simulink model "FuzzyPersonalizableDMA"  (R2024b)
settings: Solver=ode45  StartTime=0.0  StopTime=3  FixedStep=.1  RelTol=1e-3
libraries: fuzblock x1
settings Model: Creator=aceve  LastModifiedBy=david

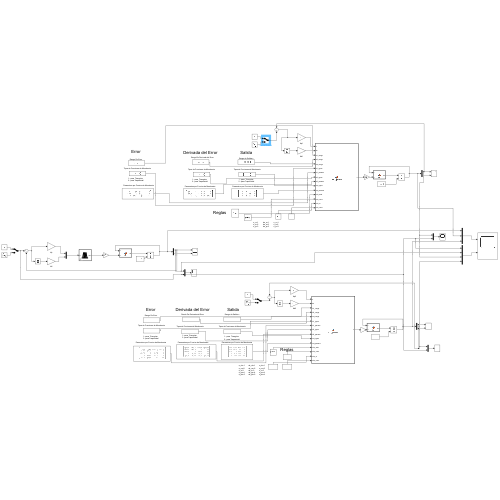
[thumbnail: Simulink's stored preview of the top-level diagram]
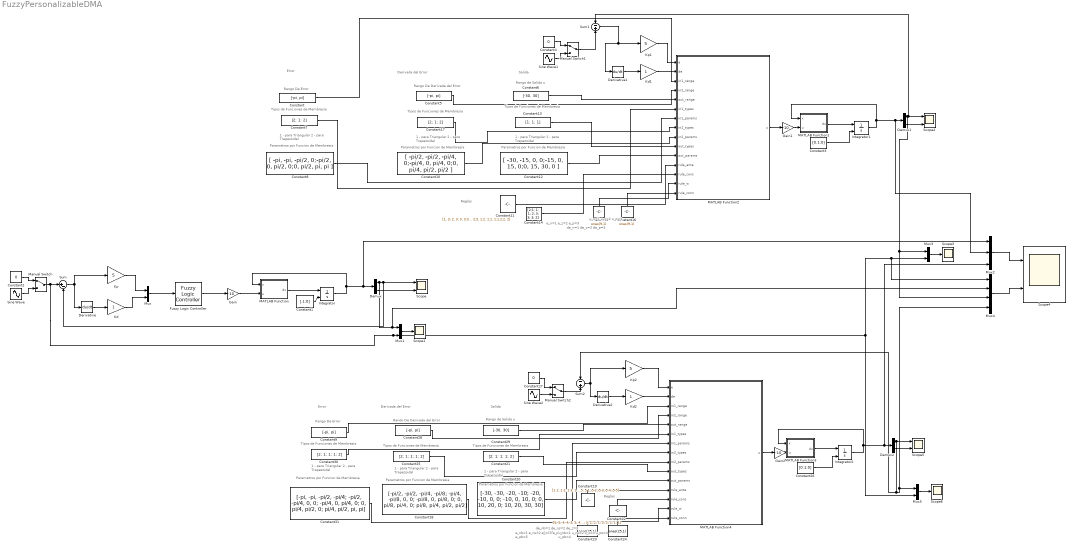
== system FuzzyPersonalizableDMA ==
  note: e_n=1
      | e_z=2
      | e_p=3
  note: Error
  note: 1 - para  Triangular
      | 2 - para Trapezoidal
  note: Parametros por Funcion de Membresia
  note: Tipos de Funciones de Membresia
  note: Rango de Salida u
  note: Rango De Derivada del Error
  note: Rango De Error
  note: 1 - para  Triangular
      | 2 - para Trapezoidal
  note: Derivada del Error
  note: Tipos de Funciones de Membresia
  note: Parametros por Funcion de Membresia
  note: 1 - para  Triangular
      | 2 - para Trapezoidal
  note: Salida
  note: Tipos de Funciones de Membresia
  note: Parametros por Funcion de Membresia
  note: Reglas
  note: de_n=1
      | de_z=2
      | de_p=3
  note: u_n=1
      | u_z=2
      | u_p=3
  note: 1 - para  Triangular
      | 2 - para Trapezoidal
  note: Tipos de Funciones de Membresia
  note: Salida
  note: de_nb=1
      | de_ns=2
      | de_z=3
      | de_ps=4
      | de_pb=5
  note: Reglas
  note: Parametros por Funcion de Membresia
  note: e_nb=1
      | e_ns=2
      | e_z=3
      | e_ps=4
      | e_pb=5
  note: Rando De Derivada del Error
  note: Error
  note: 1 - para  Triangular
      | 2 - para Trapezoidal
  note: Tipos de Funciones de Membresia
  note: Rango De Error
  note: Parametros por Funcion de Membresia
  note: Parametros por Funcion de Membresia
  note: u_nb=1
      | u_ns=2
      | u_z=3
      | u_ps=4
      | u_pb=4
  note: Tipos de Funciones de Membresia
  note: 1 - para  Triangular
      | 2 - para Trapezoidal
  note: Rango de Salida u
  note: Derivada del Error
  Constant{,5,9,28} (4 alike) : Constant  Value=[-pi, pi]
  Constant1 : Constant  Value=[.1;0]
  Constant10 : Constant  Value=[ -pi/2, -pi/2, -pi/4, 0;-pi/4, 0, pi/4, 0;0, pi/4, pi/2, pi/2 ]
  Constant11 : Constant  Value=[1, 3; 2, 3; 3, 3;3, 2;3, 1;2, 1;1, 1;1,2;2, 2]
  Constant12 : Constant  Value="[ -30, -15, 0, 0;-15,   0, 15, 0;0,  15, 30, 0 ]"
  Constant13 : Constant  Value=[1; 1; 1]
  Constant14 : Constant  Value=[2;1; 1; 1; 2; 3; 3; 3; 2]
  Constant15 : Constant  Value=ones(9,1)
  Constant16 : Constant  Value=ones(9,1)
  Constant17 : Constant  Value=[2; 1; 2]
  Constant18 : Constant  Value=[-pi/2, -pi/2, -pi/4, -pi/8; -pi/4, -pi/8, 0, 0; -pi/8, 0, pi/8, 0; 0, pi/8, pi/4, 0; pi/8, pi/4, pi/2, pi/2]
  Constant19 : Constant  Value=[1 1; 1 2; 1 3; 1 4; 1 5; 2 1; 2 2; 2 3; 2 4; 2 5; 3 1; 3 2; 3 3; 3 4; 3 5; 4 1; 4 2; 4 3; 4 4; 4 5; 5 1; 5 2; 5 3; 5 4; 5 5]
  Constant2 : Constant  Value=0
  Constant20 : Constant  Value=[-30, -30, -20, -10; -20, -10, 0, 0; -10, 0, 10, 0; 0, 10, 20, 0; 10, 20, 30, 30]
  Constant21 : Constant  Value=[2; 1; 1; 1; 2]
  Constant22 : Constant  Value=[5; 5; 4; 4; 3; 5; 4; 4; 3; 2; 4; 4; 3; 2; 2; 4; 3; 2; 2; 1; 3; 2; 2; 1; 1]
  Constant23 : Constant  Value=ones(25,1)
  Constant24 : Constant  Value=ones(25,1)
  Constant25 : Constant  Value=[2; 1; 1; 1; 2]
  Constant26 : Constant  Value=[0.1;0]
  Constant27 : Constant  Value=0
  Constant29 : Constant  Value=[-30, 30]
  Constant3 : Constant  Value=[0.1;0]
  Constant30 : Constant  Value=[2; 1; 1; 1; 2]
  Constant31 : Constant  Value=[-pi, -pi, -pi/2, -pi/4; -pi/2, -pi/4, 0, 0; -pi/4, 0, pi/4, 0; 0, pi/4, pi/2, 0; pi/4, pi/2, pi, pi]
  Constant4 : Constant  Value=0
  Constant6 : Constant  Value=[-30, 30]
  Constant7 : Constant  Value=[2; 1; 2]
  Constant8 : Constant  Value=[ -pi, -pi, -pi/2, 0;-pi/2, 0, pi/2, 0;0, pi/2, pi, pi ]
  Demux : Demux  Outputs=2
  Demux1 : Demux  Outputs=2
  Demux2 : Demux  Outputs=2
  Derivative : Derivative
  Derivative1 : Derivative
  Derivative2 : Derivative
  Fuzzy Logic Controller : fuzblock/Fuzzy Logic  Controller  FIS='3x3man.fis'  OutputSampleNumber=101  DataType=double  FuzzifiedInputs=off  RuleFiringStrengths=off  RuleOutputs=off  AggregatedOutputs=off  SimulateUsing=Interpreted execution  OutOfRangeInputValueMessage=warning  NoRuleFiredMessage=warning  EmptyOutputFuzzySetMessage=warning
  Gain : Gain  Gain=-10
  Gain1 : Gain  Gain=-10
  Gain2 : Gain  Gain=-10
  Integrator : Integrator  InitialConditionSource=external
  Integrator1 : Integrator  InitialConditionSource=external
  Integrator2 : Integrator  InitialConditionSource=external
  Kd : Gain
  Kd1 : Gain
  Kd2 : Gain
  Kp : Gain  Gain=5
  Kp1 : Gain  Gain=5
  Kp2 : Gain  Gain=5
  MATLAB Function : MATLAB Function  TreatAsAtomicUnit=on
  MATLAB Function1 : MATLAB Function  TreatAsAtomicUnit=on
  MATLAB Function2 : MATLAB Function  TreatAsAtomicUnit=on
  MATLAB Function3 : MATLAB Function  TreatAsAtomicUnit=on
  MATLAB Function4 : MATLAB Function  TreatAsAtomicUnit=on
  Manual Switch : ManualSwitch
  Manual Switch1 : ManualSwitch
  Manual Switch2 : ManualSwitch
  Mux{,1,3,5} (4 alike) : Mux  Inputs=2
  Mux2 : Mux  Inputs=3
  Mux4 : Mux
  Scope{,2,4..5} (4 alike) : Scope  NumInputPorts=2
  Scope1 : Scope
  Scope3 : Scope
  Scope6 : Scope
  Sine Wave : Sin  Amplitude=.25  Frequency=4  SampleTime=0
  Sine Wave1 : Sin  Amplitude=.25  Frequency=4  SampleTime=0
  Sine Wave2 : Sin  Amplitude=.25  Frequency=4  SampleTime=0
  Sum : Sum  Inputs=|+-
  Sum1 : Sum  Inputs=-|+
  Sum2 : Sum  Inputs=-|+
  wires:
  Integrator/1 -> MATLAB Function/1(x), Mux2/1, Demux/1
  Demux/1 -> Scope/1, Sum/2, Mux4/2, Mux1/1
  Demux/2 -> Scope/2
  Constant1/1 -> Integrator/2
  Fuzzy Logic Controller/1 -> Gain/1
  Gain/1 -> MATLAB Function/2(u)
  Mux/1 -> Fuzzy Logic Controller/1
  Kp/1 -> Mux/1
  Constant2/1 -> Manual Switch/1
  Sine Wave/1 -> Manual Switch/2
  Sum/1 -> Derivative/1, Kp/1
  Kd/1 -> Mux/2
  Derivative/1 -> Kd/1
  Mux1/1 -> Scope1/1
  MATLAB Function/1(dx) -> Integrator/1
  Sine Wave1/1 -> Manual Switch1/2
  Constant4/1 -> Manual Switch1/1
  Demux1/2 -> Scope2/2
  Demux1/1 -> Scope2/1, Sum1/1, Mux4/3, Mux3/1
  MATLAB Function1/1(dx) -> Integrator1/1
  Integrator1/1 -> MATLAB Function1/1(x), Mux2/2, Demux1/1
  Gain1/1 -> MATLAB Function1/2(u)
  Constant3/1 -> Integrator1/2
  Mux3/1 -> Scope3/1
  Derivative1/1 -> Kd1/1
  Mux2/1 -> Scope4/1
  Mux4/1 -> Scope4/2
  MATLAB Function2/1(u) -> Gain1/1
  Manual Switch1/1 -> Sum1/2
  Sum1/1 -> Derivative1/1, Kp1/1
  Constant/1 -> MATLAB Function2/3(in1_range)
  Constant5/1 -> MATLAB Function2/4(in2_range)
  Constant6/1 -> MATLAB Function2/5(out_range)
  Constant7/1 -> MATLAB Function2/6(in1_types)
  Constant8/1 -> MATLAB Function2/7(in1_params)
  Constant17/1 -> MATLAB Function2/8(in2_types)
  Constant13/1 -> MATLAB Function2/10(out_types)
  Constant12/1 -> MATLAB Function2/11(out_params)
  Manual Switch/1 -> Mux1/2, Mux5/2, Mux4/1, Mux3/2, Sum/1
  Constant16/1 -> MATLAB Function2/15(rule_conn)
  Constant15/1 -> MATLAB Function2/14(rule_w)
  Constant14/1 -> MATLAB Function2/13(rule_cons)
  Constant11/1 -> MATLAB Function2/12(rule_ante)
  Constant21/1 -> MATLAB Function4/10(out_types)
  Constant23/1 -> MATLAB Function4/14(rule_w)
  Derivative2/1 -> Kd2/1
  Constant26/1 -> Integrator2/2
  Mux5/1 -> Scope6/1
  Constant25/1 -> MATLAB Function4/8(in2_types)
  Sum2/1 -> Derivative2/1, Kp2/1
  MATLAB Function4/1(u) -> Gain2/1
  Constant9/1 -> MATLAB Function4/3(in1_range)
  Constant30/1 -> MATLAB Function4/6(in1_types)
  Manual Switch2/1 -> Sum2/2
  Gain2/1 -> MATLAB Function3/2(u)
  MATLAB Function3/1(dx) -> Integrator2/1
  Constant29/1 -> MATLAB Function4/5(out_range)
  Sine Wave2/1 -> Manual Switch2/2
  Constant22/1 -> MATLAB Function4/13(rule_cons)
  Constant18/1 -> MATLAB Function4/9(in2_params)
  Constant31/1 -> MATLAB Function4/7(in1_params)
  Integrator2/1 -> MATLAB Function3/1(x), Mux2/3, Demux2/1
  Constant24/1 -> MATLAB Function4/15(rule_conn)
  Constant19/1 -> MATLAB Function4/12(rule_ante)
  Constant20/1 -> MATLAB Function4/11(out_params)
  Demux2/1 -> Mux5/1, Mux4/4, Sum2/1, Scope5/1
  Demux2/2 -> Scope5/2
  Constant27/1 -> Manual Switch2/1
  Constant28/1 -> MATLAB Function4/4(in2_range)
  Kd2/1 -> MATLAB Function4/2(de)
  Kp2/1 -> MATLAB Function4/1(e)
  Kd1/1 -> MATLAB Function2/2(de)
  Kp1/1 -> MATLAB Function2/1(e)
  Constant10/1 -> MATLAB Function2/9(in2_params)

== matlab function FuzzyPersonalizableDMA/MATLAB Function1 ==
  data: x input; dx output; u input
function dx  = fcn(x,u)

l = 1;
m = 1;
g = 9.81;
b = 0.5;
I = m*l^2

x1 = x(1);
x2 = x(2);
dx1 = x2;
dx2 = g/l * sin(x1) - b*l/I * x2 + u/I;
dx = [dx1;dx2];

y = u;

== matlab function FuzzyPersonalizableDMA/MATLAB Function ==
  data: x input; dx output; u input
function dx  = fcn(x,u)

l = 1;
m = 1;
g = 9.81;
b = 0.5;
I = m*l^2

x1 = x(1);
x2 = x(2);
dx1 = x2;
dx2 = g/l * sin(x1) - b*l/I * x2 + u/I;
dx = [dx1;dx2];

y = u;

== matlab function FuzzyPersonalizableDMA/MATLAB Function2 ==
  data: e input; u output; de input; in1_range input; in2_range input; out_range input; in1_types input; in1_params input; in2_types input; in2_params input; out_types input; out_params input; rule_ante input; rule_cons input; rule_w input; rule_conn input
function u = FLC_generic(e, de, ...
    in1_range, in2_range, out_range, ...
    in1_types, in1_params, ...   % [N1x1], [N1x4]
    in2_types, in2_params, ...   % [N2x1], [N2x4]
    out_types, out_params, ...   % [N3x1], [N3x4]
    rule_ante, rule_cons, rule_w, rule_conn)
%#codegen
% Mamdani: AND=min, OR=max, Imp=min, Agg=max, Defuzz=centroid
% Tipos: 1=trimf (usa a,b,c en cols 1..3), 2=trapmf (usa a,b,c,d en 1..4)
% rule_ante: [R x 2] índices de MF para [e, de] (0 = "no importa")
% rule_cons: [R x 1] índice de MF de salida
% rule_w:    [R x 1] peso en [0,1]
% rule_conn: [R x 1] 1=AND(min) 2=OR(max)  (aquí solo 1 o 2)

% ---- fuzzificación entradas ----
N1 = numel(in1_types);
N2 = numel(in2_types);
muE  = zeros(1,N1);
muDE = zeros(1,N2);
for i=1:N1
    muE(i) = mf_eval(e, in1_types(i), in1_params(i,:));
end
for j=1:N2
    muDE(j) = mf_eval(de, in2_types(j), in2_params(j,:));
end

% ---- inferencia (implicación min) y agregación (max) ----
Nout = numel(out_types);
% Universo de discurso de salida
Nu = 301;
ug = linspace(out_range(1), out_range(2), Nu);
muAgg = zeros(1,Nu);

R = size(rule_ante,1);
for r = 1:R
    i = rule_ante(r,1);  % MF index para e  (0=DC)
    j = rule_ante(r,2);  % MF index para de (0=DC)
    k = rule_cons(r);    % MF index salida
    w = rule_w(r);       % peso
    conn = rule_conn(r); % 1=min, 2=max

    % firing strength del antecedente
    a1 = 1.0; if i>0, a1 = muE(i);  end
    a2 = 1.0; if j>0, a2 = muDE(j); end
    if conn==1       % AND=min
        alpha = min(a1,a2);
    else             % OR=max
        alpha = max(a1,a2);
    end
    alpha = max(0,min(1, alpha*w));

    if alpha<=0 || k<1 || k>Nout
        continue
    end

    % MF de salida recortada por alpha: mu_k_out = min(alpha, mf_out)
    mu_k = zeros(1,Nu);
    for t=1:Nu
        mu_k(t) = mf_eval(ug(t), out_types(k), out_params(k,:));
    end
    muAgg = max(muAgg, min(alpha, mu_k));
end

% ---- desdifusificación (centroide) ----
num = sum(ug .* muAgg);
den = sum(muAgg);
if den<=eps
    % sin activación: salida neutra dentro de rango
    u = 0.5*(out_range(1)+out_range(2));
else
    u = num/den;
end
end

% ================= helpers =================
function mu = mf_eval(x, type_id, p)
% p es 1x4, usa solo los necesarios
if type_id==1 % trimf [a b c]
    a=p(1); b=p(2); c=p(3);
    if x<=a || x>=c, mu=0;
    elseif x==b, mu=1;
    elseif x>a && x<b, mu=(x-a)/max(b-a,eps);
    else, mu=(c-x)/max(c-b,eps);
    end
elseif type_id==2 % trapmf [a b c d]
    a=p(1); b=p(2); c=p(3); d=p(4);
    if x<=a || x>=d, mu=0;
    elseif x>=b && x<=c, mu=1;
    elseif x>a && x<b,  mu=(x-a)/max(b-a,eps);
    else                mu=(d-x)/max(d-c,eps);
    end
else
    mu = 0; % tipo desconocido
end
end

== matlab function FuzzyPersonalizableDMA/MATLAB Function3 ==
  data: x input; dx output; u input
function dx  = fcn(x,u)

l = 1;
m = 1;
g = 9.81;
b = 0.5;
I = m*l^2

x1 = x(1);
x2 = x(2);
dx1 = x2;
dx2 = g/l * sin(x1) - b*l/I * x2 + u/I;
dx = [dx1;dx2];

y = u;

== matlab function FuzzyPersonalizableDMA/MATLAB Function4 ==
  data: e input; u output; de input; in1_range input; in2_range input; out_range input; in1_types input; in1_params input; in2_types input; in2_params input; out_types input; out_params input; rule_ante input; rule_cons input; rule_w input; rule_conn input
function u = FLC_generic(e, de, ...
    in1_range, in2_range, out_range, ...
    in1_types, in1_params, ...   % [N1x1], [N1x4]
    in2_types, in2_params, ...   % [N2x1], [N2x4]
    out_types, out_params, ...   % [N3x1], [N3x4]
    rule_ante, rule_cons, rule_w, rule_conn)
%#codegen
% Mamdani: AND=min, OR=max, Imp=min, Agg=max, Defuzz=centroid
% Tipos: 1=trimf (usa a,b,c en cols 1..3), 2=trapmf (usa a,b,c,d en 1..4)
% rule_ante: [R x 2] índices de MF para [e, de] (0 = "no importa")
% rule_cons: [R x 1] índice de MF de salida
% rule_w:    [R x 1] peso en [0,1]
% rule_conn: [R x 1] 1=AND(min) 2=OR(max)  (aquí solo 1 o 2)

% ---- fuzzificación entradas ----
N1 = numel(in1_types);
N2 = numel(in2_types);
muE  = zeros(1,N1);
muDE = zeros(1,N2);
for i=1:N1
    muE(i) = mf_eval(e, in1_types(i), in1_params(i,:));
end
for j=1:N2
    muDE(j) = mf_eval(de, in2_types(j), in2_params(j,:));
end

% ---- inferencia (implicación min) y agregación (max) ----
Nout = numel(out_types);
% Universo de discurso de salida
Nu = 301;
ug = linspace(out_range(1), out_range(2), Nu);
muAgg = zeros(1,Nu);

R = size(rule_ante,1);
for r = 1:R
    i = rule_ante(r,1);  % MF index para e  (0=DC)
    j = rule_ante(r,2);  % MF index para de (0=DC)
    k = rule_cons(r);    % MF index salida
    w = rule_w(r);       % peso
    conn = rule_conn(r); % 1=min, 2=max

    % firing strength del antecedente
    a1 = 1.0; if i>0, a1 = muE(i);  end
    a2 = 1.0; if j>0, a2 = muDE(j); end
    if conn==1       % AND=min
        alpha = min(a1,a2);
    else             % OR=max
        alpha = max(a1,a2);
    end
    alpha = max(0,min(1, alpha*w));

    if alpha<=0 || k<1 || k>Nout
        continue
    end

    % MF de salida recortada por alpha: mu_k_out = min(alpha, mf_out)
    mu_k = zeros(1,Nu);
    for t=1:Nu
        mu_k(t) = mf_eval(ug(t), out_types(k), out_params(k,:));
    end
    muAgg = max(muAgg, min(alpha, mu_k));
end

% ---- desdifusificación (centroide) ----
num = sum(ug .* muAgg);
den = sum(muAgg);
if den<=eps
    % sin activación: salida neutra dentro de rango
    u = 0.5*(out_range(1)+out_range(2));
else
    u = num/den;
end
end

% ================= helpers =================
function mu = mf_eval(x, type_id, p)
% p es 1x4, usa solo los necesarios
if type_id==1 % trimf [a b c]
    a=p(1); b=p(2); c=p(3);
    if x<=a || x>=c, mu=0;
    elseif x==b, mu=1;
    elseif x>a && x<b, mu=(x-a)/max(b-a,eps);
    else, mu=(c-x)/max(c-b,eps);
    end
elseif type_id==2 % trapmf [a b c d]
    a=p(1); b=p(2); c=p(3); d=p(4);
    if x<=a || x>=d, mu=0;
    elseif x>=b && x<=c, mu=1;
    elseif x>a && x<b,  mu=(x-a)/max(b-a,eps);
    else                mu=(d-x)/max(d-c,eps);
    end
else
    mu = 0; % tipo desconocido
end
end
